simulink model "Path_model"  (R2024b)
settings: Solver=ode1  StartTime=0.0  StopTime=30.0  FixedStep=0.5e-3  RelTol=1e-3
model workspace (MAT data in the model file):
  l = Simulink.Parameter
  l.Value = 1
  l.Complexity = 'real'
  l.Dimensions = [1 1]
  l.DataType = 'double'
settings Model: DataDictionary=Path_dd.sldd  EnableAccessToBaseWorkspace=off  ParameterArgumentNames=l  Creator=wai484  LastModifiedBy=wai484
settings SolverCC: EnableFixedStepZeroCrossing=on
settings DataIOCC: SaveOutput=off  SignalLogging=off  DSMLogging=off  StreamToWks=off  SaveTime=off  ReturnWorkspaceOutputs=off
settings OptimizationCC: DefaultParameterBehavior=Inlined  UseDivisionForNetSlopeComputation=UseDivisionForReciprocalsOfIntegersOnly  GainParamInheritBuiltInType=on  UseFloatMulNetSlope=on  InheritOutputTypeSmallerThanSingle=on  InlineInvariantSignals=on  StateBitsets=on  DataBitsets=on  EfficientFloat2IntCast=on  BufferReusableBoundary=off  SimCompilerOptimization=on  DenormalBehavior=FlushToZero
settings DebuggingCC: SignalInfNanChecking=error  SignalRangeChecking=error  ReadBeforeWriteMsg=EnableAllAsError  WriteAfterWriteMsg=EnableAllAsError  WriteAfterReadMsg=EnableAllAsError  AlgebraicLoopMsg=error  ArtificialAlgebraicLoopMsg=error  SaveWithDisabledLinksMsg=error  SaveWithParameterizedLinksMsg=error  BlockPriorityViolationMsg=error  SolverPrmCheckMsg=warning  InheritedTsInSrcMsg=error  TasksWithSamePriorityMsg=error  SigSpecEnsureSampleTimeMsg=error  CheckMatrixSingularityMsg=error  IntegerOverflowMsg=error  ParameterUnderflowMsg=error  ParameterPrecisionLossMsg=error  ParameterTunabilityLossMsg=error  UnderSpecifiedDataTypeMsg=error  UnnecessaryDatatypeConvMsg=warning  VectorMatrixConversionMsg=error  UnconnectedInputMsg=error  UnconnectedOutputMsg=error  UnconnectedLineMsg=error  SFcnCompatibilityMsg=error  UniqueDataStoreMsg=error  BusObjectLabelMismatch=error  RootOutportRequireBusObject=error  AssertControl=DisableAll  ModelReferenceIOMismatchMessage=error  UnknownTsInhSupMsg=error  ModelReferenceDataLoggingMessage=error  StateNameClashWarn=warning  StrictBusMsg=ErrorOnBusTreatedAsVector  NonBusSignalsTreatedAsBus=error  SFInvalidInputDataAccessInChartInitDiag=error  SFTransitionOutsideNaturalParentDiag=error  SFUnreachableExecutionPathDiag=error  SFUndirectedBroadcastEventsDiag=error  SFTransitionActionBeforeConditionDiag=error  SFTemporalDelaySmallerThanSampleTimeDiag=error  SFSelfTransitionDiag=error  SFExecutionAtInitializationDiag=error  IntegerSaturationMsg=error  VariantConditionMismatch=error
settings ModelReferenceCC: EnableParallelModelReferenceBuilds=on
settings SFSimCC: SimIntegrity=alwaysOn  CompileTimeRecursionLimit=0  EnableRuntimeRecursion=off  EnableImplicitExpansion=off  MATLABDynamicMemAlloc=off  SimHardwareAcceleration=native
settings RTWCC: BuildConfiguration=Faster Runs
settings GRTTargetCC: CodeReplacementLibrary=GNU C99 extensions  UtilityFuncGeneration=Shared location  CodeInterfacePackaging=Reusable function  GenerateAllocFcn=on  OptimizeReductions=on  MultiInstanceErrorCode=Warning

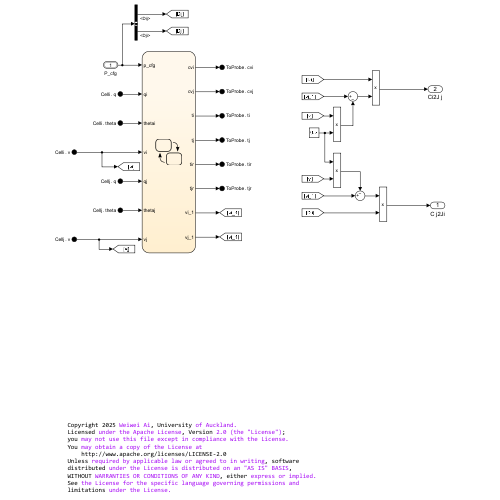
[thumbnail: Simulink's stored preview of the top-level diagram]
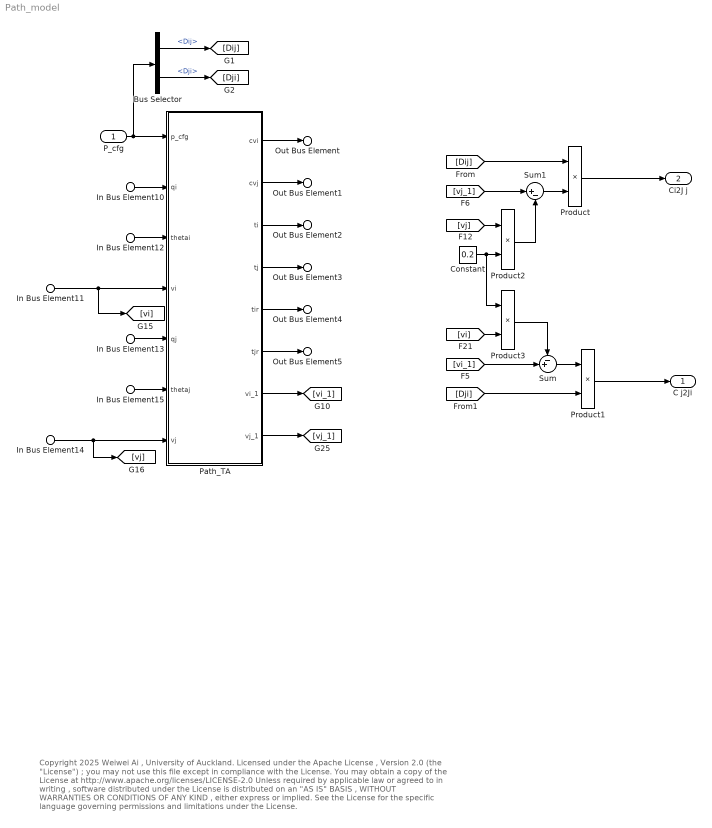
== system Path_model ==
  note: Copyright 2025 Weiwei Ai , University of Auckland.
      | Licensed under the Apache License , Version 2.0 (the "License") ;
      | you may not use this file except in compliance with the License.
      | You may obtain a copy of the License at
      | http://www.apache.org/licenses/LICENSE-2.0
      | Unless required by applicable law or agreed to in writing , software
      | distributed under the License is distributed on an "AS IS" BASIS ,
      | WITHOUT WARRANTIES OR CONDITIONS OF ANY KIND , either express or implied.
      | See the License for the specific language governing permissions and
      | limitations under the License.
  P_cfg : Inport  OutDataTypeStr=Bus: Config_Path  BusOutputAsStruct=on
  In Bus Element10 : Inport  Port=2  PortName=Celli  Element=q
  In Bus Element11 : Inport  Port=2  PortName=Celli  Element=v
  In Bus Element12 : Inport  Port=2  PortName=Celli  Element=theta
  In Bus Element13 : Inport  Port=3  PortName=Cellj  Element=q
  In Bus Element14 : Inport  Port=3  PortName=Cellj  Element=v
  In Bus Element15 : Inport  Port=3  PortName=Cellj  Element=theta
  Bus Selector : BusSelector  OutputSignals=Dij,Dji
  Constant : Constant  Value=0.2
  Path_TA : Stateflow chart  TreatAsAtomicUnit=on
  Product{,1..3} (4 alike) : Product  Inputs=**
  Sum : Sum  Inputs=-+|
  Sum1 : Sum  Inputs=|+-
  C j2Ji : Outport  OutDataTypeStr=double  PortDimensions=1  SampleTime=[0.00050000000000000001,0]
  Ci2J j : Outport  Port=2  OutDataTypeStr=double  PortDimensions=1  SampleTime=[0.00050000000000000001,0]
  Out Bus Element : Outport  Port=3  PortName=ToProbe  Element=cvi
  Out Bus Element1 : Outport  Port=3  PortName=ToProbe  Element=cvj
  Out Bus Element2 : Outport  Port=3  PortName=ToProbe  Element=ti
  Out Bus Element3 : Outport  Port=3  PortName=ToProbe  Element=tj
  Out Bus Element4 : Outport  Port=3  PortName=ToProbe  Element=tir
  Out Bus Element5 : Outport  Port=3  PortName=ToProbe  Element=tjr
  wires:
  Path_TA/8(vj_1) -> [vj_1]
  Path_TA/7(vi_1) -> [vi_1]
  [vj_1] -> Sum1/1
  Sum1/1 -> Product/2
  [vj] -> Product2/1
  Product2/1 -> Sum1/2
  Constant/1 -> Product2/2, Product3/1
  Sum/1 -> Product1/1
  Product3/1 -> Sum/1
  [vi_1] -> Sum/2
  [vi] -> Product3/2
  In Bus Element12/1 -> Path_TA/3(thetai)
  Product/1 -> Ci2J j/1
  Product1/1 -> C j2Ji/1
  In Bus Element13/1 -> Path_TA/5(qj)
  In Bus Element10/1 -> Path_TA/2(qi)
  In Bus Element15/1 -> Path_TA/6(thetaj)
  In Bus Element14/1 -> [vj], Path_TA/7(vj)
  In Bus Element11/1 -> [vi], Path_TA/4(vi)
  Path_TA/1(cvi) -> Out Bus Element/1
  Path_TA/2(cvj) -> Out Bus Element1/1
  Path_TA/6(tjr) -> Out Bus Element5/1
  Path_TA/5(tir) -> Out Bus Element4/1
  Path_TA/4(tj) -> Out Bus Element3/1
  Path_TA/3(ti) -> Out Bus Element2/1
  P_cfg/1 -> Bus Selector/1, Path_TA/1(p_cfg)
  Bus Selector/1 -> [Dij]  "<Dij>"
  Bus Selector/2 -> [Dji]  "<Dji>"
  [Dij] -> Product/1
  [Dji] -> Product1/2

== stateflow chart Path_model/Path_TA ==
  settings: updateMethod=DISCRETE
  state Wave
    state Relay_i [parallel]
      settings: executionOrder=8
      state Relay
        en: tj_1=0;
        du: tj_1=temporalCount(sec);
        vj_1=vbi(floor(tj_1)+1);
        ex: tj_1=0;
      state Idle
        en:
        vj_1=0;
      Wave.Relay_i.Idle -> Wave.Relay_i.Relay : Reach_j
      (default) -> Wave.Relay_i.Idle
      Wave.Relay_i.Relay -> Wave.Relay_i.Idle : [qj>=2 || j_1==0 ]
    state Cell_i [parallel]
      settings: executionOrder=5
      state Activation
      state Rest
        en:
        i_1=0;
      Wave.Cell_i.Rest -> Wave.Cell_i.Activation : Reach_i
      Wave.Cell_i.Activation -> Wave.Cell_i.Rest [order 1] : [after(tbj,sec)]
      (default) -> Wave.Cell_i.Rest
      Wave.Cell_i.Activation -> Wave.Cell_i.Rest [order 2] : Go_j
    state Relay_j [parallel]
      settings: executionOrder=7
      state Relay
        en: ti_1=0;
        du: ti_1=temporalCount(sec);
        vi_1=vbj(floor(ti_1)+1);
        ex: ti_1=0;
      state Idle
        en:
        vi_1=0;
      Wave.Relay_j.Idle -> Wave.Relay_j.Relay : Reach_i
      (default) -> Wave.Relay_j.Idle
      Wave.Relay_j.Relay -> Wave.Relay_j.Idle : [qi>=2 || i_1==0 ]
    state Cell_j [parallel]
      settings: executionOrder=6
      state Activation
      state Rest
        en:
        j_1=0;
      note: 1.
      Wave.Cell_j.Rest -> Wave.Cell_j.Activation : Reach_j
      Wave.Cell_j.Activation -> Wave.Cell_j.Rest [order 1] : [after(tbi,sec)]
      (default) -> Wave.Cell_j.Rest
      Wave.Cell_j.Activation -> Wave.Cell_j.Rest [order 2] : Go_i
    state End_j [parallel]
      settings: executionOrder=2
      state End_j_Idle
      state Go
        en: tj=0;
        du: tj=temporalCount(sec);
        ex: tj=0;
      note: 5
      state Ready
      note: 2.
      state BlockedByNeighbour
      Wave.End_j.Go -> Wave.End_j.End_j_Idle [order 2] : [Meet || mul==0]
      Wave.End_j.Go -> Wave.End_j.End_j_Idle [order 1] : [tj>=Tj && mul==1]
          | /{mul=mul-1;i_1=1; send(Reach_i,Cell_i);send(Reach_i,Relay_j);}
      (default) -> Wave.End_j.End_j_Idle
      Wave.End_j.End_j_Idle -> Wave.End_j.Ready [order 1] : [qj==2 && j_1==0]
      Wave.End_j.Ready -> Wave.End_j.Go [order 2] : [qj==3 && j_1==0]
          | /{ cvj=thetafcn(p_cfg.CVj2i,thetaj,p_cfg.aji,p_cfg.bji,p_cfg.cji);
          | Tj=l/cvj; mul=mul+1; send(Go_j,Buffer_j);send(Go_j,Cell_i);}
      Wave.End_j.End_j_Idle -> Wave.End_j.BlockedByNeighbour [order 2] : [qj==2 && j_1==1]
      Wave.End_j.Ready -> Wave.End_j.BlockedByNeighbour [order 1] : [cvj==0 || (qj==3 && j_1==1)]{tj=0;}
      Wave.End_j.BlockedByNeighbour -> Wave.End_j.End_j_Idle : [qj==0]
    state End_i [parallel]
      settings: executionOrder=1
      state End_i_Idle
      state Go
        en:ti=0;
        du: ti=temporalCount(sec);
        ex: ti=0;
      note: 4
      state Ready
      note: 2.
      note: 7
      state BlockedByNeighbour
      Wave.End_i.Go -> Wave.End_i.End_i_Idle [order 2] : [cvi*ti+cvj*tj>=l && mul==2]/
          | { mul=0; send(Meet,End_j);send(Meet,Buffer_i);send(Meet,Buffer_j);}
      Wave.End_i.Go -> Wave.End_i.End_i_Idle [order 1] : [ti>=Ti && mul==1]
          | /{mul=mul-1; j_1=1; send(Reach_j,Cell_j);send(Reach_j,Relay_i);}
      (default) -> Wave.End_i.End_i_Idle
      Wave.End_i.End_i_Idle -> Wave.End_i.Ready [order 1] : [qi==2 && i_1==0]
      Wave.End_i.Ready -> Wave.End_i.Go [order 2] : [qi==3 && i_1==0]
          | /{ cvi=thetafcn(p_cfg.CVi2j,thetai,p_cfg.aij,p_cfg.bij,p_cfg.cij);
          | Ti=l/cvi; mul=mul+1;send(Go_i,Buffer_i);send(Go_i,Cell_j); }
      Wave.End_i.End_i_Idle -> Wave.End_i.BlockedByNeighbour [order 2] : [qi==2 && i_1==1]
      Wave.End_i.Ready -> Wave.End_i.BlockedByNeighbour [order 1] : [cvi==0 || (qi==3 && i_1==1)]{ti=0;}
      Wave.End_i.BlockedByNeighbour -> Wave.End_i.End_i_Idle : [qi==0]
    state Buffer_i [parallel]
      settings: executionOrder=3
      state Idle
      note: 6
      state Buffer_i
        en: tbi=0;
        du: tbi=temporalCount(sec);
        vbi(floor(tbi)+1)=vi;
      (default) -> Wave.Buffer_i.Idle
      Wave.Buffer_i.Idle -> Wave.Buffer_i.Buffer_i : Go_i
      Wave.Buffer_i.Buffer_i -> Wave.Buffer_i.Idle [order 1] : [qi<3]
      Wave.Buffer_i.Buffer_i -> Wave.Buffer_i.Idle [order 2] : Meet
      Wave.Buffer_i.Buffer_i -> Wave.Buffer_i.Idle [order 3] : [tbi>=0.599]
    note: 3
    state Buffer_j [parallel]
      settings: executionOrder=4
      state Idle
      state Buffer_i
        en: tbj=0;
        du: tbj=temporalCount(sec);
        vbj(floor(tbj)+1)=vj;
      (default) -> Wave.Buffer_j.Idle
      Wave.Buffer_j.Idle -> Wave.Buffer_j.Buffer_i : Go_j
      Wave.Buffer_j.Buffer_i -> Wave.Buffer_j.Idle [order 1] : [qj<3]
      Wave.Buffer_j.Buffer_i -> Wave.Buffer_j.Idle [order 2] : Meet
      Wave.Buffer_j.Buffer_i -> Wave.Buffer_j.Idle [order 3] : [tbj>=0.599]
    state End_i_Fade [parallel]
      settings: executionOrder=10
      state End_i_Idle
      state End_i_re
        du: tir=temporalCount(sec);
      End_i_re -> Wave.End_i_Fade.End_i_Idle [order 1] : [cvi*tir+cvj*tjr>=l && tjr~=0]
          | /{send(Meet_r,End_j_Fade);tir=0;tjr=0;}
      End_i_re -> Wave.End_i_Fade.End_i_Idle [order 2] : [cvi*tir+cvj*tjr>=l&& tjr==0]/{tir=0;}
      (default) -> Wave.End_i_Fade.End_i_Idle
      Wave.End_i_Fade.End_i_Idle -> End_i_re : cell_i_r
    state End_j_Fade [parallel]
      settings: executionOrder=12
      state End_j_Idle
      state End_j_re
        du: tjr=temporalCount(sec);
      End_j_re -> Wave.End_j_Fade.End_j_Idle [order 1] : [cvi*tir+cvj*tjr>=l&& tir==0]/{tjr=0;}
      End_j_re -> Wave.End_j_Fade.End_j_Idle [order 2] : Meet_r
      (default) -> Wave.End_j_Fade.End_j_Idle
      Wave.End_j_Fade.End_j_Idle -> End_j_re : cell_j_r
    state Celll_j_Re [parallel]
      settings: executionOrder=9
      state Re
      state De
      Wave.Celll_j_Re.De -> Wave.Celll_j_Re.Re : [qj==0]/{send(cell_j_r,End_j_Fade);}
      Wave.Celll_j_Re.Re -> Wave.Celll_j_Re.De : [qj==3]
      (default) -> Wave.Celll_j_Re.Re
    state Celll_i_Re [parallel]
      settings: executionOrder=11
      state Re
      state De
      Wave.Celll_i_Re.De -> Wave.Celll_i_Re.Re : [qi==0]/{send(cell_i_r,End_i_Fade);}
      Wave.Celll_i_Re.Re -> Wave.Celll_i_Re.De : [qi==3]
      (default) -> Wave.Celll_i_Re.Re
    note: 1. The Cell_j_1 will be released if it has been resting or another AP from Cell_i starts travelling;.
    note: 2. Cell_i start to repolarize before the activation either reaches Cell_j or meets the activation from Cell_j, which happens when the APD is short or/and the path is long, e.g., premature depolarization.
        | In this case, the path would ignore all following activation before the premature activation reaches Cell_j or meets the activation from Cell_j.
  state Init
  note: 3. Assume that the APD<=600 ms; If the APD>600, it would be truncated; Store the action potential of q3 until it goes back to repolarization or meets the other one.
      | 4. j_1=1; and Reach_j must occur at the same time to block Go_j immediately;
      | 5. mul==0 to make sure the transition to take in case Meet event is missed
      | 6. qi<3 instead of qi==0 to avoid where qi==0 is missed due to the stimulation timing and the simulation step;
      | 7. when cv=0, no propagation.
  (default) -> Init
  Init -> Wave : [temporalCount(msec)>0]/{cvi=p_cfg.CVi2j;
      | cvj=p_cfg.CVj2i;
      | Ti=l/cvi;
      | Tj=l/cvj;
      | ti=0;
      | tj=0;
      | ti_1=0;
      | tj_1=0;
      | i_1=0;
      | j_1=0;
      | vi_1=0;
      | vj_1=0;
      | tir=0;
      | tjr=0;
      | tbi=0;
      | tbj=0;
      | vbi=zeros(1,600);
      | vbj=zeros(1,600);
      | mul=0;
      | }
  data: cvin function_input double; thetain function_input double; ain function_input double; bin function_input double; cin function_input double; cvout function_output double; cvi output double; cvj output double; p_cfg input Bus: Config_Path; ti output double; qi input; thetai input; vi input; qj input; thetaj input; ti_1 local double; tj_1 local double; tj output; tir output; tjr output; i_1 local; j_1 local; vi_1 output; vj_1 output; l parameter double; tbi local; tbj local; vbi local; vbj local; vj input; Ti local double; Tj local double; mul local
  events: Reach_i local FUNCTION_CALL_EVENT; Reach_j local FUNCTION_CALL_EVENT; Go_i local FUNCTION_CALL_EVENT; Go_j local FUNCTION_CALL_EVENT; Meet local FUNCTION_CALL_EVENT; Meet_r local FUNCTION_CALL_EVENT; cell_i_r local FUNCTION_CALL_EVENT; cell_j_r local FUNCTION_CALL_EVENT
  function cvout = thetafcn(cvin,thetain,ain,bin,cin):
    | function cvout = thetafcn(cvin,thetain,ain,bin,cin)
    | %#codegen
    | %Rate dependent factor
    | ftheta=1/(ain*exp(bin*thetain)+(1-ain)*exp(-cin*thetain));
    | cvout=cvin*ftheta;
    | end
